simulink model "cargadorInductivo"  (R2022b)
settings: Solver=daessc  StartTime=0.0  StopTime=1e-3  RelTol=1e-3
libraries: fl_lib x13, nesl_utility x5, spsRMSLib x4
settings Model: Creator=juanma  LastModifiedBy=juanma

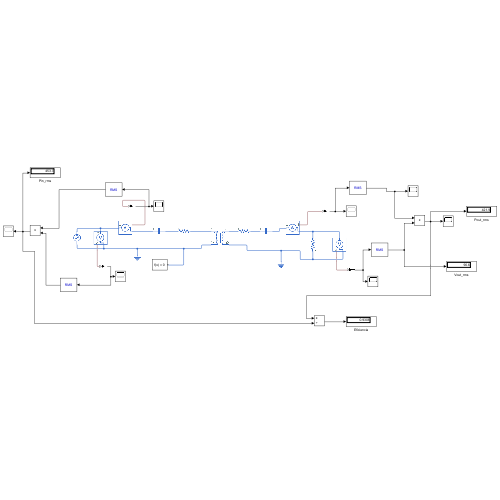
[thumbnail: Simulink's stored preview of the top-level diagram]
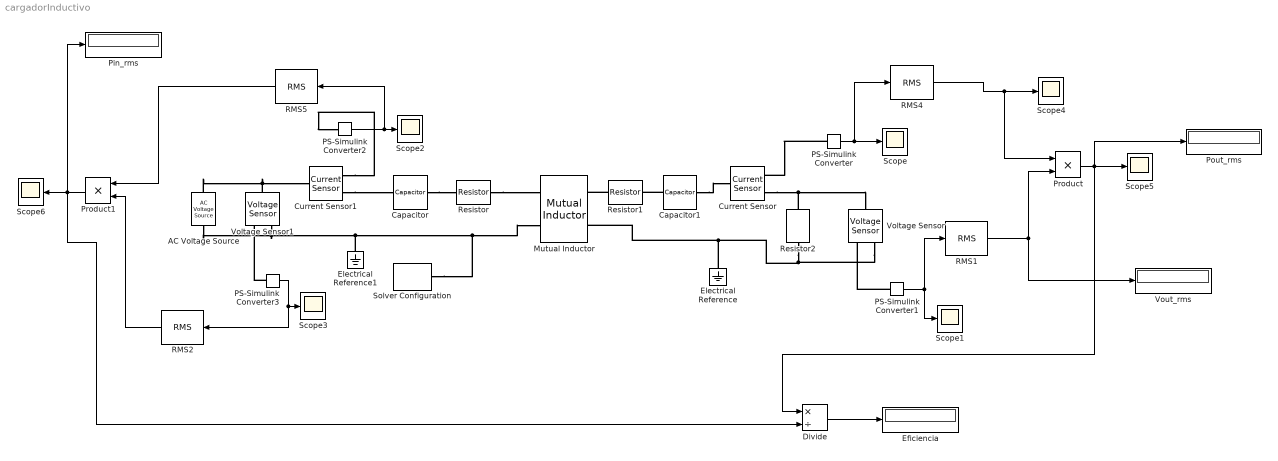
== system cargadorInductivo ==
  AC Voltage Source : fl_lib/Electrical/Electrical Sources/AC Voltage Source  amp=170 V  shift=0 deg  frequency=85 kHz  omega=0 rad/s
  Capacitor : fl_lib/Electrical/Electrical Elements/Capacitor  c=17.05 nF  r=1e-6 Ohm  g=0 1/Ohm  i_specify=off  i_priority=None  i=0 A  i_nominal_specify=off  i_nominal_unit=A  i_nominal_value=1  v_specify=off  v_priority=None  v=0 V  v_nominal_specify=off  v_nominal_unit=V  v_nominal_value=1  vc_specify=off  vc_priority=High  vc=0 V  vc_nominal_specify=off  vc_nominal_unit=V  vc_nominal_value=1
  Capacitor1 : fl_lib/Electrical/Electrical Elements/Capacitor  c=15.88 nF  r=1e-6 Ohm  g=0 1/Ohm  i_specify=off  i_priority=None  i=0 A  i_nominal_specify=off  i_nominal_unit=A  i_nominal_value=1  v_specify=off  v_priority=None  v=0 V  v_nominal_specify=off  v_nominal_unit=V  v_nominal_value=1  vc_specify=off  vc_priority=High  vc=0 V  vc_nominal_specify=off  vc_nominal_unit=V  vc_nominal_value=1
  Current Sensor : fl_lib/Electrical/Electrical Sensors/Current Sensor
  Current Sensor1 : fl_lib/Electrical/Electrical Sensors/Current Sensor
  Divide : Product  Inputs=*/
  Eficiencia : Display
  Electrical Reference : fl_lib/Electrical/Electrical Elements/Electrical Reference
  Electrical Reference1 : fl_lib/Electrical/Electrical Elements/Electrical Reference
  Mutual Inductor : fl_lib/Electrical/Electrical Elements/Mutual Inductor  L1=240.5 uH  L2=230.6 uH  k=0.2  i1_specify=off  i1_priority=High  i1=0 A  i1_nominal_specify=off  i1_nominal_unit=A  i1_nominal_value=1  i2_specify=off  i2_priority=High  i2=0 A  i2_nominal_specify=off  i2_nominal_unit=A  i2_nominal_value=1  v1_specify=off  v1_priority=None  v1=0 V  v1_nominal_specify=off  v1_nominal_unit=V  v1_nominal_value=1  v2_specify=off  v2_priority=None  v2=0 V  v2_nominal_specify=off  v2_nominal_unit=V  v2_nominal_value=1
      settings: InternalSimscapePortConfiguration="{\"Bottom\":[],\"Left\":[{\"id\":\"p1\",\"label\":\"1+\",\"type\":\"foundation.electrical.electrical\"},{\"id\":\"n1\",\"label\":\"1-\",\"type\":\"foundation.electrical.electrical\"}],\"Right\":[{\"id\":\"p2\",\"label\":\"2+\",\"type\":\"foundation.electrical.electrical\"},{\"id\":\"n2\",\"label\":\"2-\",\"type\":\"foundation.electrical.electrical\"}],\"Top\":[]}"
  PS-Simulink Converter{,1..3} (4 alike) : nesl_utility/PS-Simulink Converter  PhysicalDomain=network_engine_domain  SubClassName=ps_output  LeftPortType=input  RightPortType=output  PseudoPeriodic=off  Frequencies=[]  VectorFormat=inherit  Unit=inherit  AffineConversion=off
  Pin_rms : Display
  Pout_rms : Display
  Product : Product
  Product1 : Product
  RMS{1..2,4..5} (4 alike) : spsRMSLib/RMS  TrueRMS=off  Freq=85e3  RMSInit=0  Ts=0
  Resistor : fl_lib/Electrical/Electrical Elements/Resistor  R=195.6 mOhm  i_specify=off  i_priority=None  i=0 A  i_nominal_specify=off  i_nominal_unit=A  i_nominal_value=1  v_specify=off  v_priority=None  v=0 V  v_nominal_specify=off  v_nominal_unit=V  v_nominal_value=1
  Resistor1 : fl_lib/Electrical/Electrical Elements/Resistor  R=143.1 mOhm  i_specify=off  i_priority=None  i=0 A  i_nominal_specify=off  i_nominal_unit=A  i_nominal_value=1  v_specify=off  v_priority=None  v=0 V  v_nominal_specify=off  v_nominal_unit=V  v_nominal_value=1
  Resistor2 : fl_lib/Electrical/Electrical Elements/Resistor  R=8/(pi^2)*(240^2/2400) Ohm  i_specify=off  i_priority=None  i=0 A  i_nominal_specify=off  i_nominal_unit=A  i_nominal_value=1  v_specify=off  v_priority=None  v=0 V  v_nominal_specify=off  v_nominal_unit=V  v_nominal_value=1
  Scope{,1..6} (7 alike) : Scope
  Solver Configuration : nesl_utility/Solver Configuration  PhysicalDomain=network_engine_domain  SubClassName=solver  LeftPortType=input  RightPortType=generic  Tones=[]  Harmonics=[]  SimulateNoise=off  Profile=off  UseLocalSampling=off  EnableSwitchedLinearOptims=on  FrequencyDomain=off  UseCCode=off  RelTol=0.001  AbsTol=0.001  MinStep=1e-09  ToWorkspace=off  RevertToSquareIcSolve=off  NumHomotopyIterations=100  PhasorMode=off  PhasorModeNumHarmonics=1  ConsistencySolver=NEWTON_XTOL_AFTER_FTOL  IndexReductionMethod=DerivativeReplacement  DoDC=on  ResidualTolerance=1e-09  ConsistencyTolSource=GLOBAL  ConsistencyAbsTol=0.001  ConsistencyRelTol=0.001  ConsistencyTolFactor=0.001  UseLocalSolver=off  LocalSolverChoice=NE_BACKWARD_EULER_ADVANCER  ResolveIndetEquations=on  FunctionEvalNumThread=1  LocalSolverSampleTime=0.001  DoFixedCost=off  MaxNonlinIter=3  MaxModeIter=2  ComputeImpulses=off  ImpulseIterations=2  LinearAlgebra=auto  LinearAlgebraNumThread=0  EquationFormulation=NE_TIME_EF  DelaysMemoryBudget=1024  AutomaticFiltering=on  FilteringTimeConstant=0.001  PartitionStorageMethod=AS_NEEDED  PartitionMemoryBudget=1024  PartitionMethod=ROBUST
  Voltage Sensor : fl_lib/Electrical/Electrical Sensors/Voltage Sensor
  Voltage Sensor1 : fl_lib/Electrical/Electrical Sensors/Voltage Sensor
  Vout_rms : Display
  wires:
  PS-Simulink Converter/1 -> RMS4/1, Scope/1
  PS-Simulink Converter1/1 -> RMS1/1, Scope1/1
  PS-Simulink Converter3/1 -> RMS2/1, Scope3/1
  RMS4/1 -> Product/1, Scope4/1
  RMS1/1 -> Product/2, Vout_rms/1
  Product/1 -> Divide/1, Pout_rms/1, Scope5/1
  RMS2/1 -> Product1/2
  PS-Simulink Converter2/1 -> RMS5/1, Scope2/1
  Product1/1 -> Divide/2, Pin_rms/1, Scope6/1
  RMS5/1 -> Product1/1
  Divide/1 -> Eficiencia/1
  connections:
  Resistor/RConn1 -- Mutual Inductor/LConn1
  AC Voltage Source/RConn1 -- Voltage Sensor1/RConn2 -- Electrical Reference1/LConn1 -- Solver Configuration/RConn1 -- Mutual Inductor/LConn2
  Resistor1/LConn1 -- Mutual Inductor/RConn1
  Resistor2/RConn1 -- Voltage Sensor/RConn2 -- Electrical Reference/LConn1 -- Mutual Inductor/RConn2
  Resistor2/LConn1 -- Current Sensor/RConn2 -- Voltage Sensor/LConn1
  PS-Simulink Converter/LConn1 -- Current Sensor/RConn1
  PS-Simulink Converter1/LConn1 -- Voltage Sensor/RConn1
  Capacitor/RConn1 -- Resistor/LConn1
  Capacitor1/LConn1 -- Resistor1/RConn1
  Capacitor1/RConn1 -- Current Sensor/LConn1
  Current Sensor1/RConn2 -- Capacitor/LConn1
  Voltage Sensor1/LConn1 -- Current Sensor1/LConn1 -- AC Voltage Source/LConn1
  PS-Simulink Converter3/LConn1 -- Voltage Sensor1/RConn1
  Current Sensor1/RConn1 -- PS-Simulink Converter2/LConn1
